simulink model "uavQ_H_PID_Validation"  (R2024a)
settings: Solver=ode113  StartTime=0.0  StopTime=20  FixedStep=0.01  RelTol=1e-3  EnableMultiTasking=on
values from neighbouring files (symbols this model uses):
  along = [-0.0709051452518 -0.0312761201157 3.64057642679e-14 0 0 2.85492242454 -5.43216735908 -43.1077767614 0 -24.9999999995 -3.77183093786e-12 0.999999999997 ... (25 elements, 5x5)]    [data.mat]    (also in uavck_0.3ma.mat = [-0.0324066456698 -0.0020163512714 -0.000626412946339 0 -4.3)
  blong = [-8.21411807948e-14  0.0245045555074; -0.00768014371519  -4.00476593595e-05; -0.804098256542  0; 0  0; 0  0]    [data.mat]    (also in uavck_0.3ma.mat = [-0.0673606939615  3.97585187094; -0.00795176637424  -0.0012)
  clong = [1 0 0 0 0 0 57.2957795131 0 0 0 0 0 ... (25 elements, 5x5)]    [data.mat]    (also in uavck_0.3ma.mat = [0.999999999996 0 0 0 0 0 57.2957804904 0 0 0 0 0 ... (25 el)
  dlong = [0  0; 0  0; 0  0; 0  0; 0  0]    [data.mat]    (also in uavck_0.3ma.mat)
  utrim = [-0.27394440066 -2.18120400277e-14 2.66036165513e-14 36.1693692171]    [data.mat]    (also in uavck_0.3ma.mat = [3.01593434862 -3.12927644793e-17 -4.76262648152e-17 0.40338)
  ytrim = [25 2.3396530782 1.37911498271e-14 -1.7963177274e-14 -1.87974334034e-13 100.031205124 -4.04263501627e-21 1.15674010744e-20 -9.76571062923e-22 -2.660361454e-14 2.3396530782 0 ... (13 elements, 13x1)]    [data.mat]    (also in uavck_0.3ma.mat = [100.930378182 3.74826362454 -1.61286790598e-16 4.7626264815)
settings Model: Creator=Administrator  LastModifiedBy=rzxha
settings SolverCC: AlgebraicLoopSolver=TrustRegion
settings DataIOCC: SaveFormat=Array  SignalLoggingSaveFormat=ModelDataLogs  ReturnWorkspaceOutputs=off  SignalLoggingName=sigsOut
settings OptimizationCC: BooleanDataType=off  ExpressionDepthLimit=2147483647  InitFltsAndDblsToZero=on  LifeSpan=inf
settings DebuggingCC: SaveWithParameterizedLinksMsg=none  UnderspecifiedInitializationDetection=Classic  MergeDetectMultiDrivingBlocksExec=none  SignalResolutionControl=TryResolveAllWithWarning  MultiTaskDSMMsg=warning  MultiTaskCondExecSysMsg=none  FcnCallInpInsideContextMsg=warning  UnconnectedInputMsg=warning  UnconnectedOutputMsg=warning  UnconnectedLineMsg=warning  StateNameClashWarn=warning  SFUnexpectedBacktrackingDiag=warning  SFNoUnconditionalDefaultTransitionDiag=warning  ArithmeticOperatorsInVariantConditions=warning
settings HardwareCC: ProdBitPerPointer=32  ProdBitPerSizeT=32  ProdBitPerPtrDiffT=32  ProdLargestAtomicFloat=None  ProdIntDivRoundTo=Undefined  ProdEndianess=Unspecified  ProdWordSize=32  ProdHWDeviceType=32-bit Generic  TargetUnknown=on
settings ModelReferenceCC: EnableRefExpFcnMdlSchedulingChecks=on  PropagateSignalLabelsOutOfModel=off
settings SFSimCC: SimUseLocalCustomCode=off  CustomCodeUndefinedFunction=UseInterfaceOnly
settings RTWCC: RTWUseLocalCustomCode=off  GPUComputeCapability=3.5
settings CodeAppCC: StateflowObjectComments=on
settings GRTTargetCC: TargetFcnLib=ansi_tfl_tmw.mat  TargetLangStandard=C89/C90 (ANSI)  CombineOutputUpdateFcns=off  GRTInterface=on
settings ConfigComp: CovMetricSettings=dw  CovSaveCumulativeToWorkspaceVar=on  CovSaveSingleToWorkspaceVar=on  CovExternalEMLEnable=off

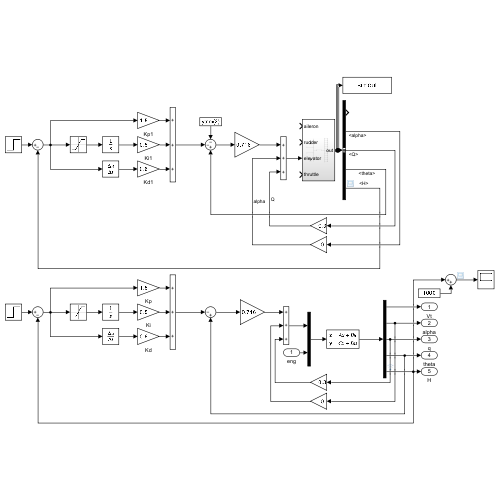
[thumbnail: Simulink's stored preview of the top-level diagram]
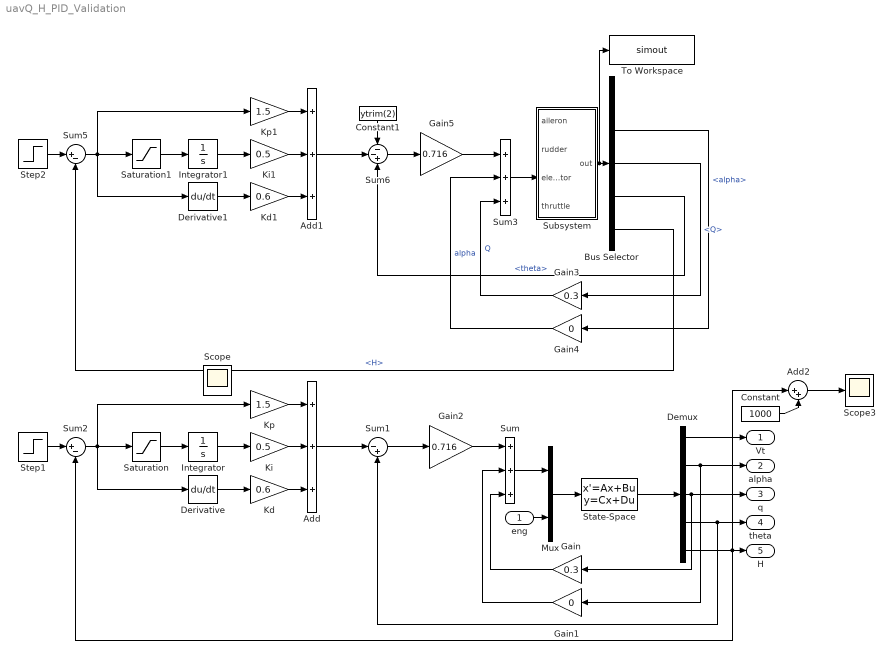
== system uavQ_H_PID_Validation ==
  eng : Inport
  Add : Sum  Inputs=+++
  Add1 : Sum  Inputs=+++
  Add2 : Sum  Inputs=|++
  Bus Selector : BusSelector  OutputSignals=Vt,alpha,Q,theta,H
  Constant : Constant  Value=1000
  Constant1 : Constant  Value=ytrim(2)
  Demux : Demux  Outputs=5
  Derivative : Derivative
  Derivative1 : Derivative
  Gain : Gain  Gain=0.3
  Gain1 : Gain  Gain=0
  Gain2 : Gain  Gain=0.716
  Gain3 : Gain  Gain=0.3
  Gain4 : Gain  Gain=0
  Gain5 : Gain  Gain=0.716
  Integrator : Integrator
  Integrator1 : Integrator
  Kd : Gain  Gain=0.6
  Kd1 : Gain  Gain=0.6
  Ki : Gain  Gain=0.5
  Ki1 : Gain  Gain=0.5
  Kp : Gain  Gain=1.5
  Kp1 : Gain  Gain=1.5
  Mux : Mux  Inputs=2
  Saturation : Saturate
  Saturation1 : Saturate
  Scope3 : Scope
  State-Space : StateSpace  A=along  B=blong  C=clong  D=dlong  InitialCondition=[0 rad2deg(0) 0 rad2deg(0) 0]
  Step1 : Step  SampleTime=0
  Step2 : Step  Before=1000  After=1001  SampleTime=0
  Subsystem : Subsystem
  Sum : Sum  Inputs=+++
  Sum1 : Sum  Inputs=|-+
  Sum2 : Sum  Inputs=|+-
  Sum3 : Sum  Inputs=+++
  Sum5 : Sum  Inputs=|+-
  Sum6 : Sum  Inputs=--+
  To Workspace : ToWorkspace  VariableName=simout  SaveFormat=Timeseries  SampleTime=-1
  Vt : Outport  VectorParamsAs1DForOutWhenUnconnected=off
  alpha : Outport  Port=2  VectorParamsAs1DForOutWhenUnconnected=off
  q : Outport  Port=3  VectorParamsAs1DForOutWhenUnconnected=off
  theta : Outport  Port=4  VectorParamsAs1DForOutWhenUnconnected=off
  H : Outport  Port=5  VectorParamsAs1DForOutWhenUnconnected=off
  Scope : Scope
  wires:
  Demux/1 -> Vt/1
  Demux/3 -> q/1, Gain/1
  Demux/4 -> theta/1, Sum1/2
  Demux/5 -> Add2/1, H/1, Sum2/2
  Demux/2 -> alpha/1, Gain1/1
  State-Space/1 -> Demux/1
  Mux/1 -> State-Space/1
  Sum1/1 -> Gain2/1
  Sum/1 -> Mux/1
  Gain/1 -> Sum/3
  Gain1/1 -> Sum/2
  Gain2/1 -> Sum/1
  Integrator/1 -> Ki/1
  Derivative/1 -> Kd/1
  Saturation/1 -> Integrator/1
  Kp/1 -> Add/1
  Ki/1 -> Add/2
  Kd/1 -> Add/3
  Sum2/1 -> Saturation/1, Kp/1, Derivative/1
  Step1/1 -> Sum2/1
  Add/1 -> Sum1/1
  Bus Selector/5 -> Sum5/2  "<H>"
  Step2/1 -> Sum5/1
  Sum5/1 -> Saturation1/1, Kp1/1, Derivative1/1
  Kp1/1 -> Add1/1
  Gain3/1 -> Sum3/3  "Q"
  Saturation1/1 -> Integrator1/1
  Integrator1/1 -> Ki1/1
  Kd1/1 -> Add1/3
  Ki1/1 -> Add1/2
  Gain4/1 -> Sum3/2  "alpha"
  Sum6/1 -> Gain5/1
  Derivative1/1 -> Kd1/1
  Bus Selector/3 -> Gain3/1  "<Q>"
  Bus Selector/4 -> Sum6/3  "<theta>"
  Bus Selector/2 -> Gain4/1  "<alpha>"
  eng/1 -> Mux/2
  Constant/1 -> Add2/2
  Add2/1 -> Scope3/1
  Sum3/1 -> Subsystem/3(elevator)
  Add1/1 -> Sum6/2
  Constant1/1 -> Sum6/1
  Gain5/1 -> Sum3/1
  Subsystem/1(out) -> Bus Selector/1, To Workspace/1

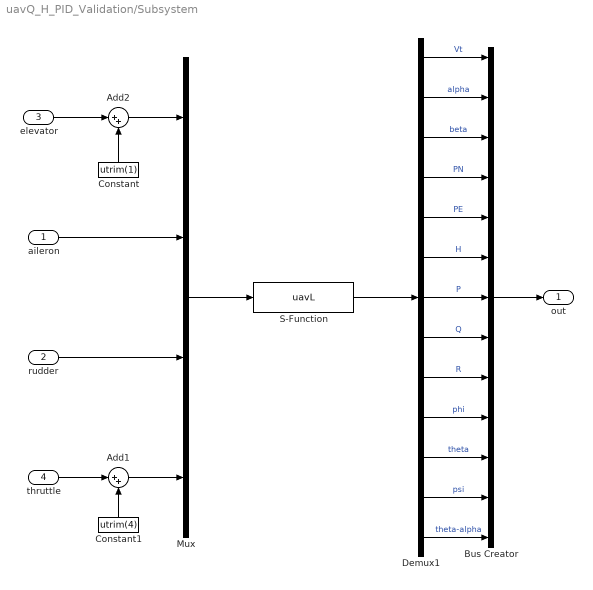
== system uavQ_H_PID_Validation/Subsystem ==
  aileron : Inport
  rudder : Inport  Port=2
  elevator : Inport  Port=3
  thruttle : Inport  Port=4
  Add1 : Sum  Inputs=|++
  Add2 : Sum  Inputs=|++
  Bus Creator : BusCreator  Inputs=13
  Constant : Constant  Value=utrim(1)
  Constant1 : Constant  Value=utrim(4)
  Demux1 : Demux  Outputs=13
  Mux : Mux
  S-Function : S-Function  FunctionName=uavL  SFunctionDeploymentMode=off  EnableBusSupport=off
  out : Outport
  wires:
  Add1/1 -> Mux/4
  thruttle/1 -> Add1/1
  Constant1/1 -> Add1/2
  rudder/1 -> Mux/3
  Demux1/4 -> Bus Creator/4  "PN"
  Add2/1 -> Mux/1
  Mux/1 -> S-Function/1
  Constant/1 -> Add2/2
  aileron/1 -> Mux/2
  elevator/1 -> Add2/1
  Demux1/11 -> Bus Creator/11  "theta"
  S-Function/1 -> Demux1/1
  Demux1/12 -> Bus Creator/12  "psi"
  Demux1/5 -> Bus Creator/5  "PE"
  Demux1/10 -> Bus Creator/10  "phi"
  Demux1/6 -> Bus Creator/6  "H"
  Demux1/2 -> Bus Creator/2  "alpha"
  Demux1/1 -> Bus Creator/1  "Vt"
  Demux1/3 -> Bus Creator/3  "beta"
  Demux1/13 -> Bus Creator/13  "theta-alpha"
  Demux1/9 -> Bus Creator/9  "R"
  Demux1/8 -> Bus Creator/8  "Q"
  Demux1/7 -> Bus Creator/7  "P"
  Bus Creator/1 -> out/1
